simulink model "lab6_sim"  (R2022b)
settings: Solver=VariableStepAuto  StartTime=0.0  StopTime=czas_symulacji  RelTol=1e-3
values from neighbouring files (symbols this model uses):
  Cvp = cp*ro*Vp    (= 36000)    [lab5_modyfikacja.m]    (also in lab6.m; lab7.m)
  Cvw = cp*ro*Vw    (= 72000)    [lab5_modyfikacja.m]    (also in lab6.m; lab7.m)
  dqg = 0.1*qgN    (= 1000)    [lab5_modyfikacja.m]    (also in lab6.m; lab7.m)
  dTzew = 0    [lab5_modyfikacja.m]    (also in lab6.m; lab7.m)
  Kcp = (a*Kcw*(TwewN-TpN))/(TpN-TzewN)    (= 26.8199233716)    [Lab2.m]    (also in lab5_modyfikacja.m; lab6.m; lab7.m)
  Kcw = qgN/((TwewN-TzewN)+a*(TwewN-TpN))    (= 229.885057471)    [Lab2.m]    (also in lab5_modyfikacja.m; lab6.m; lab7.m)
  Kcwp = (Kcp*(TpN-TzewN))/(TwewN-TpN)    (= 80.4597701149)    [Lab2.m]    (also in lab5_modyfikacja.m; lab6.m; lab7.m)
  L11 = [Cvp (Kcwp+Kcp)]    [lab5_modyfikacja.m]    (also in lab6.m = 0.004; lab7.m = 0.004)
  L12 = [Cvp*Kcw (Kcw*(Kcwp+Kcp)+Kcwp*Kcp)]    [lab5_modyfikacja.m]    (also in lab6.m = 0.003; lab7.m = 0.003)
  M11 = [T_w 1]    [lab6.m]    (also in lab7.m)
  M12 = [T_p 1]    [lab6.m]    (also in lab7.m)
  qg0 = 0:0.1*qgN:qgN    [Lab2.m]    (also in lab5_modyfikacja.m = [qgN qgN qgN*zmiana_qg]; lab6.m = 0; lab7.m = 10000)
  t0 = 1000    [lab5_modyfikacja.m]    (also in lab6.m; lab7.m)
  T0p = 1050    [lab6.m]    (also in lab7.m = 1060)
  T0w = 1000    [lab6.m]    (also in lab7.m)
  Tp0 = ((a*Kcw*Twew0)+Kcp*Tzew0)/(a*Kcw+Kcp)    [Lab2.m]    (also in lab5_modyfikacja.m; lab6.m = 0; lab7.m = 10)
  TpN = 10    [Lab2.m]    (also in lab5_modyfikacja.m; lab6.m; lab7.m)
  Twew0 = (qg(i)*(a*Kcw+Kcp)+Tzew0*(Kcw*(a*Kcw+Kcp)+(a*Kcw*Kcp)))/(Kcw*(a*Kcw+Kcp)+a*Kcw*Kcp)    [Lab2.m]    (also in lab5_modyfikacja.m = (qg0*(a*Kcw+Kcp)+Tzew0*(Kcw*(a*Kcw+Kcp)+(a*Kcw*Kcp)))/(Kcw*(; lab6.m = 0; lab7.m = 20)
  TwewN = 20    [Lab2.m]    (also in lab5_modyfikacja.m; lab6.m; lab7.m)
  Tzew0 = -20:20    [Lab2.m]    (also in lab5_modyfikacja.m = [TzewN TzewN+zmiana_Tzew TzewN]; lab6.m = 0; lab7.m = -20)
settings Model: Creator=kubab  LastModifiedBy=kubab
settings DataIOCC: ReturnWorkspaceOutputs=off

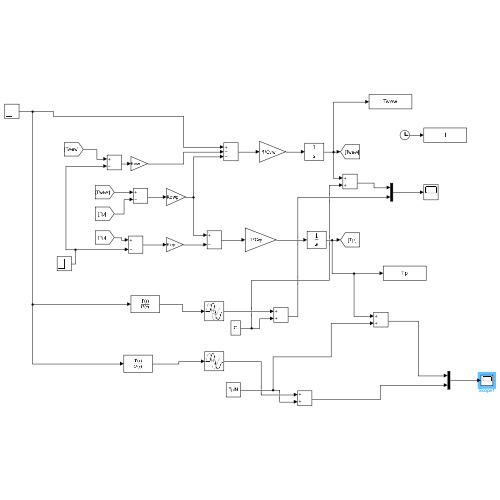
[thumbnail: Simulink's stored preview of the top-level diagram]
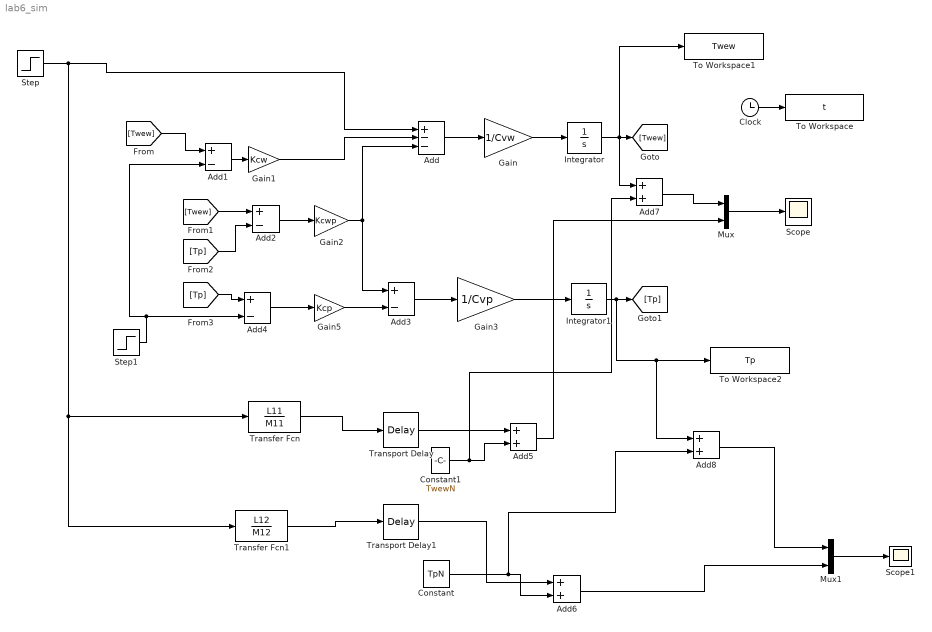
== system lab6_sim ==
  Add : Sum  Inputs=+--
  Add{1..4} (4 alike) : Sum  Inputs=+-
  Add{5..8} (4 alike) : Sum
  Clock : Clock
  Constant : Constant  Value=TpN
  Constant1 : Constant  Value=TwewN
  Gain : Gain  Gain=1/Cvw
  Gain1 : Gain  Gain=Kcw
  Gain2 : Gain  Gain=Kcwp
  Gain3 : Gain  Gain=1/Cvp
  Gain5 : Gain  Gain=Kcp
  Integrator : Integrator  InitialCondition=Twew0
  Integrator1 : Integrator  InitialCondition=Tp0
  Mux : Mux  Inputs=2
  Mux1 : Mux  Inputs=2
  Scope : Scope
  Scope1 : Scope
  Step : Step  Time=t0  Before=qg0  After=qg0+dqg  SampleTime=0
  Step1 : Step  Time=t0  Before=Tzew0  After=Tzew0+dTzew  SampleTime=0
  To Workspace : ToWorkspace  VariableName=t  SaveFormat=Timeseries  SampleTime=-1
  To Workspace1 : ToWorkspace  VariableName=Twew  SampleTime=-1
  To Workspace2 : ToWorkspace  VariableName=Tp  SampleTime=-1
  Transfer Fcn : TransferFcn  Numerator=L11  Denominator=M11
  Transfer Fcn1 : TransferFcn  Numerator=L12  Denominator=M12
  Transport Delay : TransportDelay  DelayTime=T0w
  Transport Delay1 : TransportDelay  DelayTime=T0p
  wires:
  Step/1 -> Transfer Fcn1/1, Transfer Fcn/1, Add/1
  Mux/1 -> Scope/1
  Gain/1 -> Integrator/1
  Mux1/1 -> Scope1/1
  Transfer Fcn1/1 -> Transport Delay1/1
  Gain2/1 -> Add3/1, Add/3
  [Tp] -> Add4/1
  Clock/1 -> To Workspace/1
  Add/1 -> Gain/1
  Add4/1 -> Gain5/1
  Transfer Fcn/1 -> Transport Delay/1
  Gain1/1 -> Add/2
  Add2/1 -> Gain2/1
  Step1/1 -> Add4/2, Add1/2
  [Tp] -> Add2/2
  Integrator/1 -> Add7/1, To Workspace1/1, [Twew]
  Add3/1 -> Gain3/1
  Gain3/1 -> Integrator1/1
  Integrator1/1 -> Add8/1, To Workspace2/1, [Tp]
  [Twew] -> Add1/1
  Gain5/1 -> Add3/2
  [Twew] -> Add2/1
  Add1/1 -> Gain1/1
  Transport Delay1/1 -> Add6/1
  Transport Delay/1 -> Add5/1
  Add5/1 -> Mux/2
  Add6/1 -> Mux1/2
  Constant1/1 -> Add7/2, Add5/2
  Constant/1 -> Add8/2, Add6/2
  Add7/1 -> Mux/1
  Add8/1 -> Mux1/1
